simulink model "modele"  (R2025b)
settings: Solver=VariableStepAuto  StartTime=0.0  StopTime=20  RelTol=1e-3
values from neighbouring files (symbols this model uses):
  K = 1    [mySTksi.m]    (also in variables.m)
  Np = 1e-10    [variables.m]
  Ts = 0.01    [variables.m]
  w_n = 1    [variables.m]
libraries: simulink x2, sharedTrackingLibrary x1
settings Model: Creator=flo  LastModifiedBy=flo

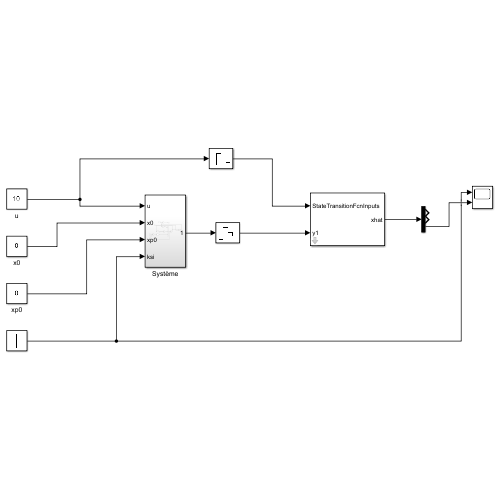
[thumbnail: Simulink's stored preview of the top-level diagram]
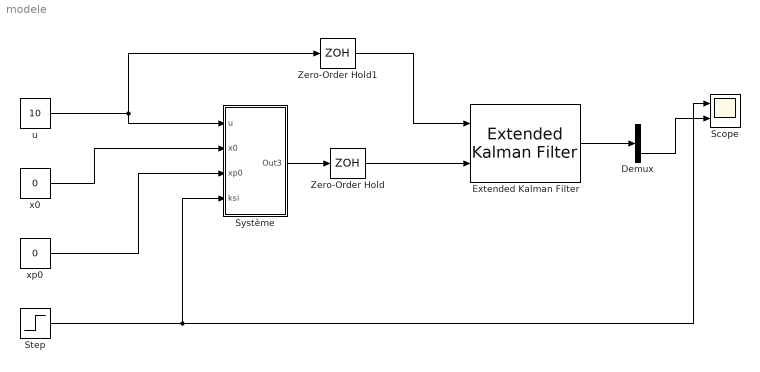
== system modele ==
  Demux : Demux  Outputs=3
  Extended Kalman Filter : sharedTrackingLibrary/Extended Kalman Filter  StateTransitionFcn=mySTksi  HasStateTransitionJacobianFcn=off  HasAdditiveProcessNoise=Additive  ProcessNoise=Qf  HasTimeVaryingProcessNoise=off  HasStateTransitionFcnExtraArgument=1  InitialState=x_init  InitialStateCovariance=1  MeasurementFcn1=myMksi  HasMeasurementJacobianFcn1=off  HasMeasurementEnablePort1=off  HasAdditiveMeasurementNoise1=Additive  MeasurementNoise1=Rf  HasTimeVaryingMeasurementNoise1=off  HasMeasurementFcnExtraArgument1=0  HasMeasurementWrapping1=off  MeasurementFcn2=myMeasurementFcn  HasMeasurementJacobianFcn2=off  HasMeasurementEnablePort2=off  HasAdditiveMeasurementNoise2=Additive  MeasurementNoise2=1  HasTimeVaryingMeasurementNoise2=off  HasMeasurementFcnExtraArgument2=0  HasMeasurementWrapping2=off  MeasurementFcn3=myMeasurementFcn  HasMeasurementJacobianFcn3=off  HasMeasurementEnablePort3=off  HasAdditiveMeasurementNoise3=Additive  MeasurementNoise3=1  HasTimeVaryingMeasurementNoise3=off  HasMeasurementFcnExtraArgument3=0  HasMeasurementWrapping3=off  MeasurementFcn4=myMeasurementFcn  HasMeasurementJacobianFcn4=off  HasMeasurementEnablePort4=off  HasAdditiveMeasurementNoise4=Additive  MeasurementNoise4=1  HasTimeVaryingMeasurementNoise4=off  HasMeasurementFcnExtraArgument4=0  HasMeasurementWrapping4=off  MeasurementFcn5=myMeasurementFcn  HasMeasurementJacobianFcn5=off  HasMeasurementEnablePort5=off  HasAdditiveMeasurementNoise5=Additive  MeasurementNoise5=1  HasTimeVaryingMeasurementNoise5=off  HasMeasurementFcnExtraArgument5=0  HasMeasurementWrapping5=off  EnableMultirate=off  StateTransitionFcnSampleTime=1  MeasurementFcn1SampleTime=1  MeasurementFcn2SampleTime=1  MeasurementFcn3SampleTime=1  MeasurementFcn4SampleTime=1  MeasurementFcn5SampleTime=1  UseCurrentEstimator=on  OutputStateCovariance=off  DataType=double  SampleTime=Ts  NumberOfMeasurements=1
  Scope : Scope  NumInputPorts=2
      settings: ActiveDisplayYMinimum=0.060204191004633804  ActiveDisplayYMaximum=0.45545335427004024
  Step : Step  Time=10  Before=0.2  After=0.4  SampleTime=0
  Système : Subsystem
  Zero-Order Hold : ZeroOrderHold  SampleTime=Ts
  Zero-Order Hold1 : ZeroOrderHold  SampleTime=Ts
  u : Constant  Value=10
  x0 : Constant  Value=0
  xp0 : Constant  Value=0
  wires:
  Système/1(Out3) -> Zero-Order Hold/1
  u/1 -> Système/1(u), Zero-Order Hold1/1
  xp0/1 -> Système/3(xp0)
  x0/1 -> Système/2(x0)
  Zero-Order Hold/1 -> Extended Kalman Filter/2
  Step/1 -> Scope/1, Système/4(ksi)
  Extended Kalman Filter/1 -> Demux/1
  Demux/3 -> Scope/2
  Zero-Order Hold1/1 -> Extended Kalman Filter/1

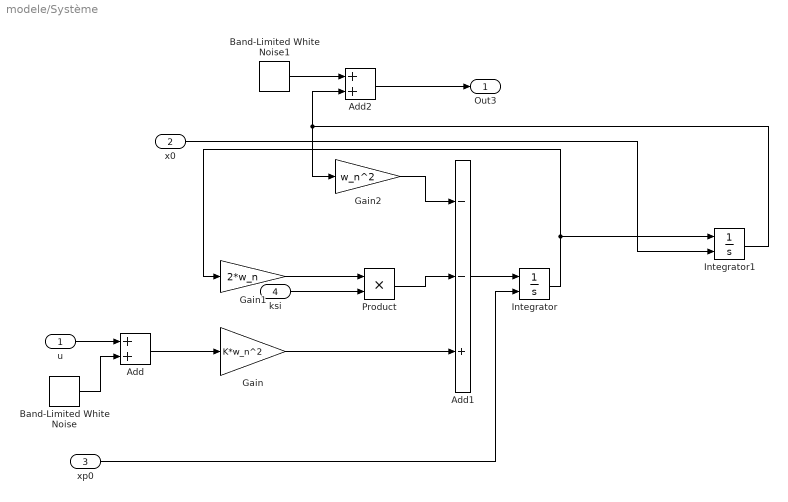
== system modele/Système ==
  u : Inport
  x0 : Inport  Port=2
  xp0 : Inport  Port=3
  ksi : Inport  Port=4
  Add : Sum
  Add1 : Sum  Inputs=--+
  Add2 : Sum
  Band-Limited White Noise : simulink/Sources/Band-Limited White Noise  Cov=[Np]  Ts=Ts  seed=[23341]
  Band-Limited White Noise1 : simulink/Sources/Band-Limited White Noise  Cov=[Np]  Ts=Ts  seed=[23341]
  Gain : Gain  Gain=K*w_n^2
  Gain1 : Gain  Gain=2*w_n
  Gain2 : Gain  Gain=w_n^2
  Integrator : Integrator  InitialConditionSource=external
  Integrator1 : Integrator  InitialConditionSource=external
  Product : Product
  Out3 : Outport
  wires:
  Add2/1 -> Out3/1
  Add/1 -> Gain/1
  Integrator/1 -> Integrator1/1, Gain1/1
  Integrator1/1 -> Gain2/1, Add2/2
  xp0/1 -> Integrator/2
  Product/1 -> Add1/2
  Gain1/1 -> Product/1
  Gain2/1 -> Add1/1
  u/1 -> Add/1
  Add1/1 -> Integrator/1
  Band-Limited White Noise/1 -> Add/2
  x0/1 -> Integrator1/2
  Gain/1 -> Add1/3
  Band-Limited White Noise1/1 -> Add2/1
  ksi/1 -> Product/2
